simulink model "Decen_control"  (R2022a)
settings: Solver=FixedStepAuto  StartTime=0.0  StopTime=10  FixedStep=Ts  RelTol=1e-3
undefined symbols (not defined in the file): duration, effort, IFV, index, joint_name, LF_body2thigh, LF_thigh2calf, LH_body2thigh, LH_thigh2calf, model_name, RF_body2thigh, RF_thigh2calf, RH_body2thigh, RH_thigh2calf
libraries: robotgazebolib x27
settings Model: PauseTimes=2  Creator=liltrump  LastModifiedBy=liltrump

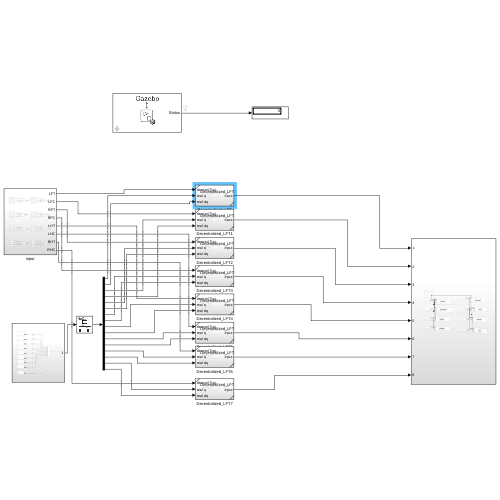
[thumbnail: Simulink's stored preview of the top-level diagram]
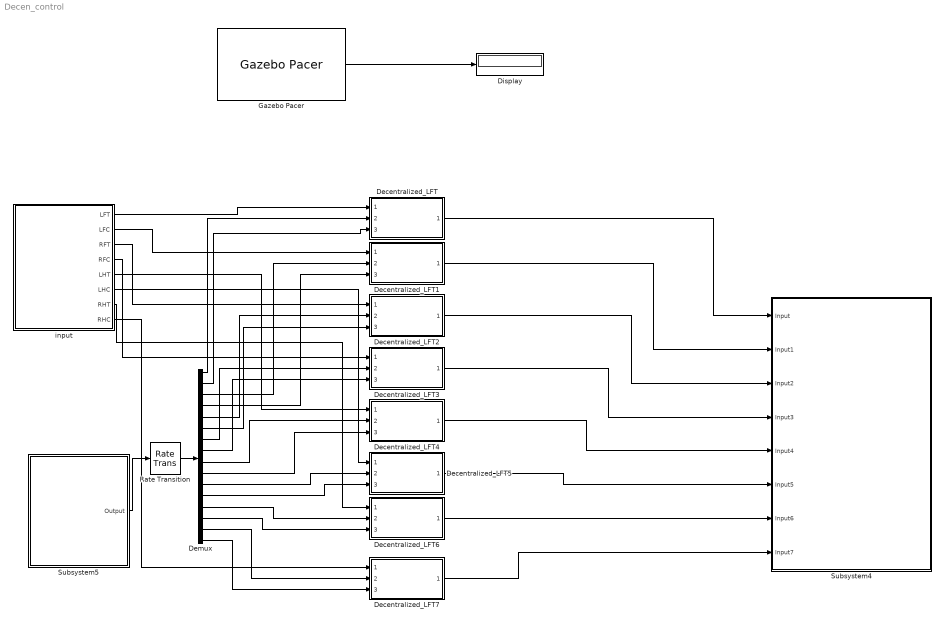
== system Decen_control ==
  Decentralized_LFT{,1..7} (8 alike) : Subsystem  VariantControl=Choice  ReferencedSubsystem=Decentralized_LFT
  Demux : Demux  Outputs=16
  Display : Display
  Gazebo Pacer : robotgazebolib/Gazebo Pacer  ResetBehavior=Reset Gazebo simulation time and scene  SampleTime=0.001
      settings: SourceProductBaseCode=RO
  Rate Transition : RateTransition  OutPortSampleTimeOpt=Inherit
  Subsystem4 : Subsystem
  Subsystem5 : Subsystem
  input : Subsystem
  wires:
  Gazebo Pacer/1 -> Display/1
  Subsystem5/1(Output) -> Rate Transition/1
  Decentralized_LFT1/1 -> Subsystem4/2(Input1)
  Decentralized_LFT2/1 -> Subsystem4/3(Input2)
  Decentralized_LFT3/1 -> Subsystem4/4(Input3)
  Decentralized_LFT4/1 -> Subsystem4/5(Input4)
  Decentralized_LFT5/1 -> Subsystem4/6(Input5)
  Decentralized_LFT6/1 -> Subsystem4/7(Input6)
  Decentralized_LFT7/1 -> Subsystem4/8(Input7)
  Demux/3 -> Decentralized_LFT1/2
  Demux/4 -> Decentralized_LFT1/3
  Demux/5 -> Decentralized_LFT2/2
  Demux/6 -> Decentralized_LFT2/3
  Demux/7 -> Decentralized_LFT3/2
  Demux/8 -> Decentralized_LFT3/3
  Demux/9 -> Decentralized_LFT4/2
  Demux/10 -> Decentralized_LFT4/3
  Demux/11 -> Decentralized_LFT5/2
  Demux/12 -> Decentralized_LFT5/3
  Demux/13 -> Decentralized_LFT6/2
  Demux/14 -> Decentralized_LFT6/3
  Demux/15 -> Decentralized_LFT7/2
  Demux/16 -> Decentralized_LFT7/3
  input/2(LFC) -> Decentralized_LFT1/1
  input/3(RFT) -> Decentralized_LFT2/1
  input/4(RFC) -> Decentralized_LFT3/1
  input/5(LHT) -> Decentralized_LFT4/1
  input/6(LHC) -> Decentralized_LFT5/1
  input/7(RHT) -> Decentralized_LFT6/1
  input/8(RHC) -> Decentralized_LFT7/1
  Rate Transition/1 -> Demux/1
  input/1(LFT) -> Decentralized_LFT/1
  Demux/1 -> Decentralized_LFT/2
  Demux/2 -> Decentralized_LFT/3
  Decentralized_LFT/1 -> Subsystem4/1(Input)

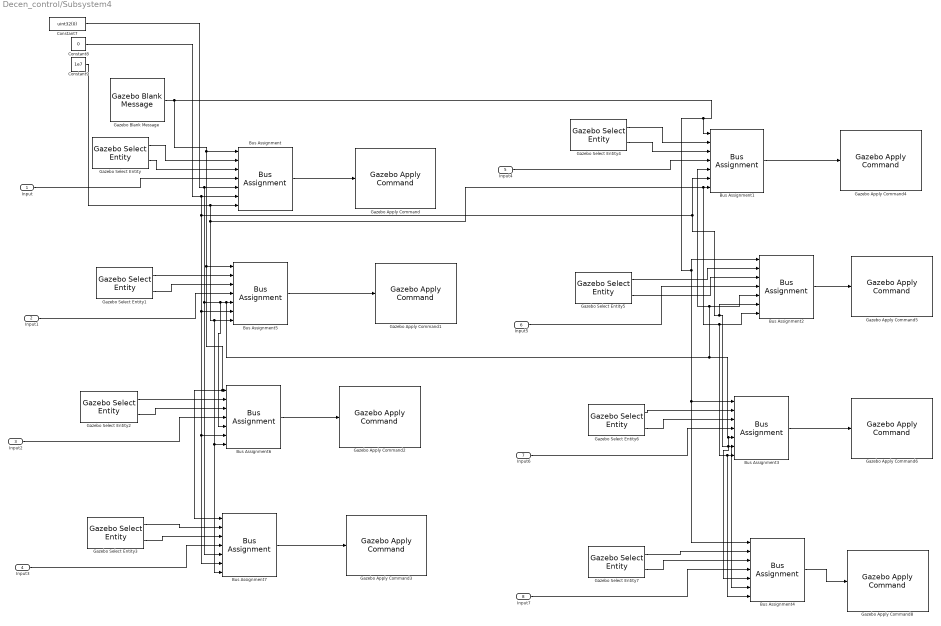
== system Decen_control/Subsystem4 ==
  Input : Inport
  Input1 : Inport  Port=2
  Input2 : Inport  Port=3
  Input3 : Inport  Port=4
  Input4 : Inport  Port=5
  Input5 : Inport  Port=6
  Input6 : Inport  Port=7
  Input7 : Inport  Port=8
  Bus Assignment{,1..7} (8 alike) : BusAssignment  AssignedSignals=model_name,joint_name,effort,index,duration.seconds,duration.nano_seconds
  Constant7 : Constant  Value=uint32(0)
  Constant8 : Constant  Value=0
  Constant9 : Constant  Value=1e7
  Gazebo Apply Command{,1..6,8} (8 alike) : robotgazebolib/Gazebo Apply Command  cmdType=ApplyJointTorque  sampleTime=0.001
      settings: SourceProductBaseCode=RO
  Gazebo Blank Message : robotgazebolib/Gazebo Blank Message  msgType=ApplyJointTorque  sampleTime=0.001  busName='Gazebo_SL_Bus_gazebo_msgs_ApplyJointTorque'
      settings: SourceProductBaseCode=RO
  Gazebo Select Entity : robotgazebolib/Gazebo Select Entity  modelElemName=IFV/LF_body2thigh  outputArraySize=128  OutputLabel=Joint  SelectType=Joint
      settings: SourceProductBaseCode=RO
  Gazebo Select Entity1 : robotgazebolib/Gazebo Select Entity  modelElemName=IFV/LF_thigh2calf  outputArraySize=128  OutputLabel=Joint  SelectType=Joint
      settings: SourceProductBaseCode=RO
  Gazebo Select Entity2 : robotgazebolib/Gazebo Select Entity  modelElemName=IFV/RF_body2thigh  outputArraySize=128  OutputLabel=Joint  SelectType=Joint
      settings: SourceProductBaseCode=RO
  Gazebo Select Entity3 : robotgazebolib/Gazebo Select Entity  modelElemName=IFV/RF_thigh2calf  outputArraySize=128  OutputLabel=Joint  SelectType=Joint
      settings: SourceProductBaseCode=RO
  Gazebo Select Entity4 : robotgazebolib/Gazebo Select Entity  modelElemName=IFV/LH_body2thigh  outputArraySize=128  OutputLabel=Joint  SelectType=Joint
      settings: SourceProductBaseCode=RO
  Gazebo Select Entity5 : robotgazebolib/Gazebo Select Entity  modelElemName=IFV/LH_thigh2calf  outputArraySize=128  OutputLabel=Joint  SelectType=Joint
      settings: SourceProductBaseCode=RO
  Gazebo Select Entity6 : robotgazebolib/Gazebo Select Entity  modelElemName=IFV/RH_body2thigh  outputArraySize=128  OutputLabel=Joint  SelectType=Joint
      settings: SourceProductBaseCode=RO
  Gazebo Select Entity7 : robotgazebolib/Gazebo Select Entity  modelElemName=IFV/RH_thigh2calf  outputArraySize=128  OutputLabel=Joint  SelectType=Joint
      settings: SourceProductBaseCode=RO
  wires:
  Gazebo Select Entity/1 -> Bus Assignment/2
  Bus Assignment/1 -> Gazebo Apply Command/1
  Bus Assignment5/1 -> Gazebo Apply Command1/1
  Input1/1 -> Bus Assignment5/4
  Gazebo Select Entity1/1 -> Bus Assignment5/2
  Gazebo Select Entity1/2 -> Bus Assignment5/3
  Bus Assignment6/1 -> Gazebo Apply Command2/1
  Input2/1 -> Bus Assignment6/4
  Gazebo Select Entity2/1 -> Bus Assignment6/2
  Gazebo Select Entity2/2 -> Bus Assignment6/3
  Bus Assignment7/1 -> Gazebo Apply Command3/1
  Input3/1 -> Bus Assignment7/4
  Gazebo Select Entity3/1 -> Bus Assignment7/2
  Gazebo Select Entity3/2 -> Bus Assignment7/3
  Bus Assignment1/1 -> Gazebo Apply Command4/1
  Gazebo Select Entity4/1 -> Bus Assignment1/2
  Gazebo Select Entity4/2 -> Bus Assignment1/3
  Bus Assignment2/1 -> Gazebo Apply Command5/1
  Gazebo Select Entity5/1 -> Bus Assignment2/2
  Gazebo Select Entity5/2 -> Bus Assignment2/3
  Bus Assignment3/1 -> Gazebo Apply Command6/1
  Input6/1 -> Bus Assignment3/4
  Gazebo Select Entity6/1 -> Bus Assignment3/2
  Gazebo Select Entity6/2 -> Bus Assignment3/3
  Bus Assignment4/1 -> Gazebo Apply Command8/1
  Input7/1 -> Bus Assignment4/4
  Gazebo Select Entity7/1 -> Bus Assignment4/2
  Gazebo Blank Message/1 -> Bus Assignment1/1, Bus Assignment2/1, Bus Assignment4/1, Bus Assignment3/1, Bus Assignment5/1, Bus Assignment7/1, Bus Assignment6/1, Bus Assignment/1
  Gazebo Select Entity7/2 -> Bus Assignment4/3
  Constant7/1 -> Bus Assignment/5, Bus Assignment6/5, Bus Assignment4/5, Bus Assignment3/5, Bus Assignment1/5, Bus Assignment2/5, Bus Assignment5/5, Bus Assignment7/5
  Constant8/1 -> Bus Assignment7/6, Bus Assignment6/6, Bus Assignment5/6, Bus Assignment4/6, Bus Assignment3/6, Bus Assignment2/6, Bus Assignment1/6, Bus Assignment/6
  Constant9/1 -> Bus Assignment5/7, Bus Assignment7/7, Bus Assignment6/7, Bus Assignment4/7, Bus Assignment3/7, Bus Assignment2/7, Bus Assignment1/7, Bus Assignment/7
  Input4/1 -> Bus Assignment1/4
  Input5/1 -> Bus Assignment2/4
  Input/1 -> Bus Assignment/4
  Gazebo Select Entity/2 -> Bus Assignment/3

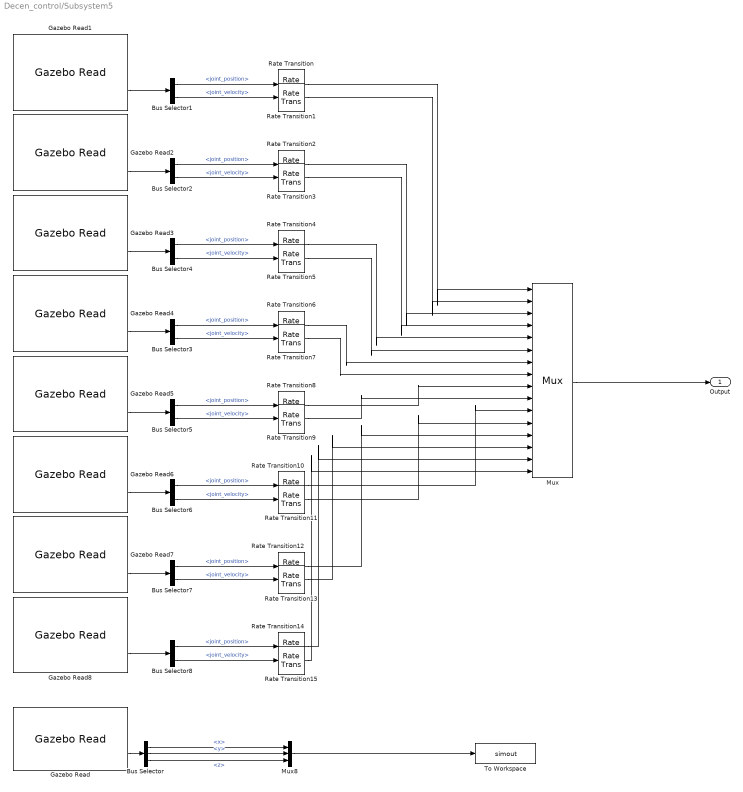
== system Decen_control/Subsystem5 ==
  Bus Selector : BusSelector  OutputSignals=world_linear_velocity.x,world_linear_velocity.y,world_linear_velocity.z
  Bus Selector{1..8} (8 alike) : BusSelector  OutputSignals=joint_position,joint_velocity
  Gazebo Read : robotgazebolib/Gazebo Read  topicSource=From Gazebo  topic=/gazebo/ground_truth/link_state/IFV/chassis  messageType=gazebo_msgs/LinkState  sampleTime=0.001
      settings: SourceProductBaseCode=RO
  Gazebo Read1 : robotgazebolib/Gazebo Read  topicSource=From Gazebo  topic=/gazebo/ground_truth/joint_state/IFV/LF_body2thigh  messageType=gazebo_msgs/JointState  sampleTime=0.001
      settings: SourceProductBaseCode=RO
  Gazebo Read2 : robotgazebolib/Gazebo Read  topicSource=From Gazebo  topic=/gazebo/ground_truth/joint_state/IFV/LF_thigh2calf  messageType=gazebo_msgs/JointState  sampleTime=0.001
      settings: SourceProductBaseCode=RO
  Gazebo Read3 : robotgazebolib/Gazebo Read  topicSource=From Gazebo  topic=/gazebo/ground_truth/joint_state/IFV/RF_body2thigh  messageType=gazebo_msgs/JointState  sampleTime=0.001
      settings: SourceProductBaseCode=RO
  Gazebo Read4 : robotgazebolib/Gazebo Read  topicSource=From Gazebo  topic=/gazebo/ground_truth/joint_state/IFV/RF_thigh2calf  messageType=gazebo_msgs/JointState  sampleTime=0.001
      settings: SourceProductBaseCode=RO
  Gazebo Read5 : robotgazebolib/Gazebo Read  topicSource=From Gazebo  topic=/gazebo/ground_truth/joint_state/IFV/LH_body2thigh  messageType=gazebo_msgs/JointState  sampleTime=0.001
      settings: SourceProductBaseCode=RO
  Gazebo Read6 : robotgazebolib/Gazebo Read  topicSource=From Gazebo  topic=/gazebo/ground_truth/joint_state/IFV/LH_thigh2calf  messageType=gazebo_msgs/JointState  sampleTime=0.001
      settings: SourceProductBaseCode=RO
  Gazebo Read7 : robotgazebolib/Gazebo Read  topicSource=From Gazebo  topic=/gazebo/ground_truth/joint_state/IFV/RH_body2thigh  messageType=gazebo_msgs/JointState  sampleTime=0.001
      settings: SourceProductBaseCode=RO
  Gazebo Read8 : robotgazebolib/Gazebo Read  topicSource=From Gazebo  topic=/gazebo/ground_truth/joint_state/IFV/RH_thigh2calf  messageType=gazebo_msgs/JointState  sampleTime=0.001
      settings: SourceProductBaseCode=RO
  Mux : Mux  Inputs=16
  Mux8 : Mux  Inputs=3
  Rate Transition{,1..15} (16 alike) : RateTransition
  To Workspace : ToWorkspace  VariableName=simout  SaveFormat=Timeseries  SampleTime=-1
  Output : Outport
  wires:
  Mux8/1 -> To Workspace/1
  Gazebo Read1/2 -> Bus Selector1/1
  Gazebo Read2/2 -> Bus Selector2/1
  Gazebo Read4/2 -> Bus Selector3/1
  Gazebo Read3/2 -> Bus Selector4/1
  Gazebo Read5/2 -> Bus Selector5/1
  Gazebo Read6/2 -> Bus Selector6/1
  Gazebo Read7/2 -> Bus Selector7/1
  Gazebo Read8/2 -> Bus Selector8/1
  Bus Selector1/1 -> Rate Transition/1  "<joint_position>"
  Bus Selector1/2 -> Rate Transition1/1  "<joint_velocity>"
  Bus Selector2/1 -> Rate Transition2/1  "<joint_position>"
  Bus Selector2/2 -> Rate Transition3/1  "<joint_velocity>"
  Bus Selector4/1 -> Rate Transition4/1  "<joint_position>"
  Bus Selector4/2 -> Rate Transition5/1  "<joint_velocity>"
  Bus Selector3/1 -> Rate Transition6/1  "<joint_position>"
  Bus Selector3/2 -> Rate Transition7/1  "<joint_velocity>"
  Bus Selector5/1 -> Rate Transition8/1  "<joint_position>"
  Bus Selector5/2 -> Rate Transition9/1  "<joint_velocity>"
  Bus Selector6/1 -> Rate Transition10/1  "<joint_position>"
  Bus Selector6/2 -> Rate Transition11/1  "<joint_velocity>"
  Bus Selector7/1 -> Rate Transition12/1  "<joint_position>"
  Bus Selector7/2 -> Rate Transition13/1  "<joint_velocity>"
  Bus Selector8/1 -> Rate Transition14/1  "<joint_position>"
  Bus Selector8/2 -> Rate Transition15/1  "<joint_velocity>"
  Rate Transition/1 -> Mux/1
  Rate Transition1/1 -> Mux/2
  Rate Transition2/1 -> Mux/3
  Rate Transition3/1 -> Mux/4
  Rate Transition4/1 -> Mux/5
  Rate Transition5/1 -> Mux/6
  Rate Transition6/1 -> Mux/7
  Rate Transition7/1 -> Mux/8
  Rate Transition8/1 -> Mux/9
  Rate Transition9/1 -> Mux/10
  Rate Transition10/1 -> Mux/11
  Rate Transition11/1 -> Mux/12
  Rate Transition12/1 -> Mux/13
  Rate Transition13/1 -> Mux/14
  Rate Transition14/1 -> Mux/15
  Rate Transition15/1 -> Mux/16
  Mux/1 -> Output/1
  Gazebo Read/2 -> Bus Selector/1
  Bus Selector/1 -> Mux8/1  "<x>"
  Bus Selector/2 -> Mux8/2  "<y>"
  Bus Selector/3 -> Mux8/3  "<z>"

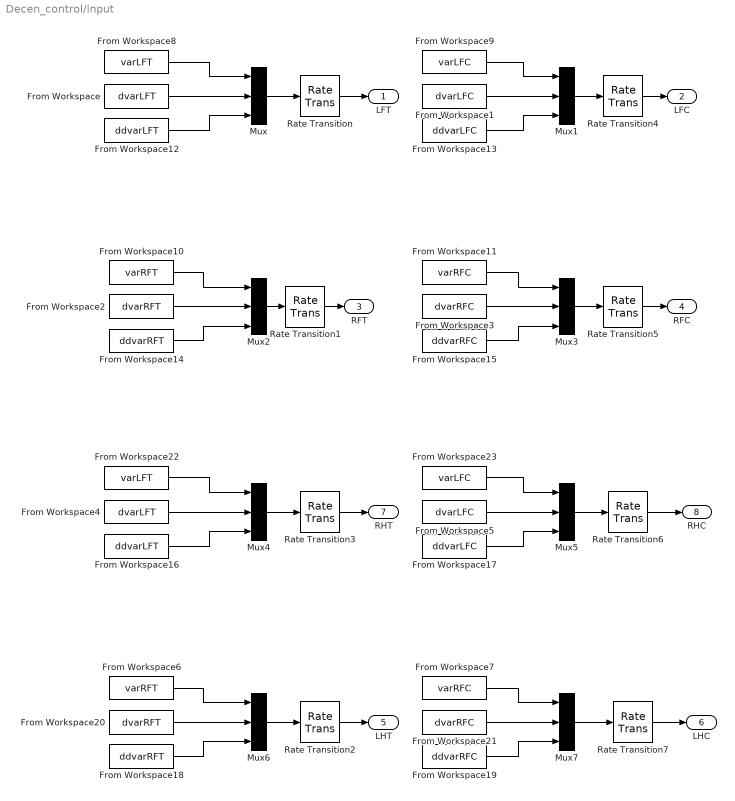
== system Decen_control/input ==
  From Workspace : FromWorkspace  VariableName=dvarLFT
  From Workspace1 : FromWorkspace  VariableName=dvarLFC
  From Workspace10 : FromWorkspace  VariableName=varRFT
  From Workspace11 : FromWorkspace  VariableName=varRFC
  From Workspace12 : FromWorkspace  VariableName=ddvarLFT
  From Workspace13 : FromWorkspace  VariableName=ddvarLFC
  From Workspace14 : FromWorkspace  VariableName=ddvarRFT
  From Workspace15 : FromWorkspace  VariableName=ddvarRFC
  From Workspace16 : FromWorkspace  VariableName=ddvarLFT
  From Workspace17 : FromWorkspace  VariableName=ddvarLFC
  From Workspace18 : FromWorkspace  VariableName=ddvarRFT
  From Workspace19 : FromWorkspace  VariableName=ddvarRFC
  From Workspace2 : FromWorkspace  VariableName=dvarRFT
  From Workspace20 : FromWorkspace  VariableName=dvarRFT
  From Workspace21 : FromWorkspace  VariableName=dvarRFC
  From Workspace22 : FromWorkspace  VariableName=varLFT
  From Workspace23 : FromWorkspace  VariableName=varLFC
  From Workspace3 : FromWorkspace  VariableName=dvarRFC
  From Workspace4 : FromWorkspace  VariableName=dvarLFT
  From Workspace5 : FromWorkspace  VariableName=dvarLFC
  From Workspace6 : FromWorkspace  VariableName=varRFT
  From Workspace7 : FromWorkspace  VariableName=varRFC
  From Workspace8 : FromWorkspace  VariableName=varLFT  OutputAfterFinalValue=Setting to zero
  From Workspace9 : FromWorkspace  VariableName=varLFC
  Mux{,1..7} (8 alike) : Mux  Inputs=3
  Rate Transition{,1..7} (8 alike) : RateTransition
  LFT : Outport
  LFC : Outport  Port=2
  RFT : Outport  Port=3
  RFC : Outport  Port=4
  LHT : Outport  Port=5
  LHC : Outport  Port=6
  RHT : Outport  Port=7
  RHC : Outport  Port=8
  wires:
  From Workspace8/1 -> Mux/1
  From Workspace/1 -> Mux/2
  From Workspace12/1 -> Mux/3
  From Workspace10/1 -> Mux2/1
  From Workspace2/1 -> Mux2/2
  From Workspace14/1 -> Mux2/3
  From Workspace9/1 -> Mux1/1
  From Workspace1/1 -> Mux1/2
  From Workspace13/1 -> Mux1/3
  From Workspace11/1 -> Mux3/1
  From Workspace3/1 -> Mux3/2
  From Workspace15/1 -> Mux3/3
  Mux1/1 -> Rate Transition4/1
  Mux2/1 -> Rate Transition1/1
  Mux3/1 -> Rate Transition5/1
  From Workspace6/1 -> Mux6/1
  From Workspace19/1 -> Mux7/3
  From Workspace20/1 -> Mux6/2
  Mux4/1 -> Rate Transition3/1
  From Workspace5/1 -> Mux5/2
  From Workspace17/1 -> Mux5/3
  From Workspace21/1 -> Mux7/2
  From Workspace22/1 -> Mux4/1
  Mux5/1 -> Rate Transition6/1
  From Workspace18/1 -> Mux6/3
  From Workspace23/1 -> Mux5/1
  From Workspace16/1 -> Mux4/3
  Mux7/1 -> Rate Transition7/1
  Mux6/1 -> Rate Transition2/1
  From Workspace7/1 -> Mux7/1
  From Workspace4/1 -> Mux4/2
  Mux/1 -> Rate Transition/1
  Rate Transition/1 -> LFT/1
  Rate Transition1/1 -> RFT/1
  Rate Transition2/1 -> LHT/1
  Rate Transition3/1 -> RHT/1
  Rate Transition4/1 -> LFC/1
  Rate Transition5/1 -> RFC/1
  Rate Transition6/1 -> RHC/1
  Rate Transition7/1 -> LHC/1
